simulink model "bandpass_eq"  (R2023a)
settings: Solver=FixedStepDiscrete  StartTime=0.0  StopTime=simParams.stopTime  RelTol=1e-3
PostLoadFcn:
  | postLoadCallback
InitFcn:
  | initCallback
StopFcn:
  | stopCallback
values from neighbouring files (symbols this model uses):
  modelParams = createFFTFilters(modelParams)    [createModelParams.m]
libraries: hdlsllib x13, dspsrcs4 x7, simulink x7, dsphdlxfrm2 x2, dspsigops x1
CloseFcn:
  | closeCallback
settings Model: DataTypeOverride=Off  Creator=Ross  LastModifiedBy=Antho
settings SolverCC: AlgebraicLoopSolver=TrustRegion
settings DataIOCC: ReturnWorkspaceOutputs=off
settings OptimizationCC: BlockReduction=off  ConditionallyExecuteInputs=off  DefaultParameterBehavior=Inlined  InheritOutputTypeSmallerThanSingle=on
settings DebuggingCC: ReadBeforeWriteMsg=DisableAll  WriteAfterWriteMsg=DisableAll  WriteAfterReadMsg=DisableAll  AlgebraicLoopMsg=error  MultiTaskDSMMsg=none  SingleTaskRateTransMsg=error  UnconnectedInputMsg=warning  UnconnectedOutputMsg=warning  UnconnectedLineMsg=warning  PregeneratedLibrarySubsystemCodeDiagnostic=none  ArithmeticOperatorsInVariantConditions=warning
settings HardwareCC: ProdBitPerPointer=32  ProdBitPerSizeT=32  ProdBitPerPtrDiffT=32  ProdLargestAtomicFloat=None  ProdIntDivRoundTo=Undefined  ProdEndianess=Unspecified  ProdWordSize=32  ProdHWDeviceType=ASIC/FPGA->ASIC/FPGA  TargetBitPerPointer=64  TargetBitPerSizeT=64  TargetBitPerPtrDiffT=64  TargetLongLongMode=on  TargetIntDivRoundTo=Zero  TargetEndianess=LittleEndian  TargetWordSize=64  TargetHWDeviceType=Custom Processor->MATLAB Host Computer  ProdEqTarget=off
settings ModelReferenceCC: UpdateModelReferenceTargets=IfOutOfDate  EnableRefExpFcnMdlSchedulingChecks=on
settings SFSimCC: SFSimEcho=off  SimUseLocalCustomCode=off  CustomCodeUndefinedFunction=UseInterfaceOnly
settings RTWCC: RTWUseLocalCustomCode=off  DLArmComputeVersion=19.05

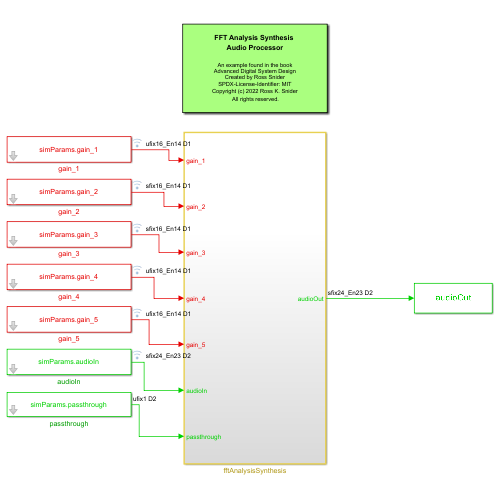
[thumbnail: Simulink's stored preview of the top-level diagram]
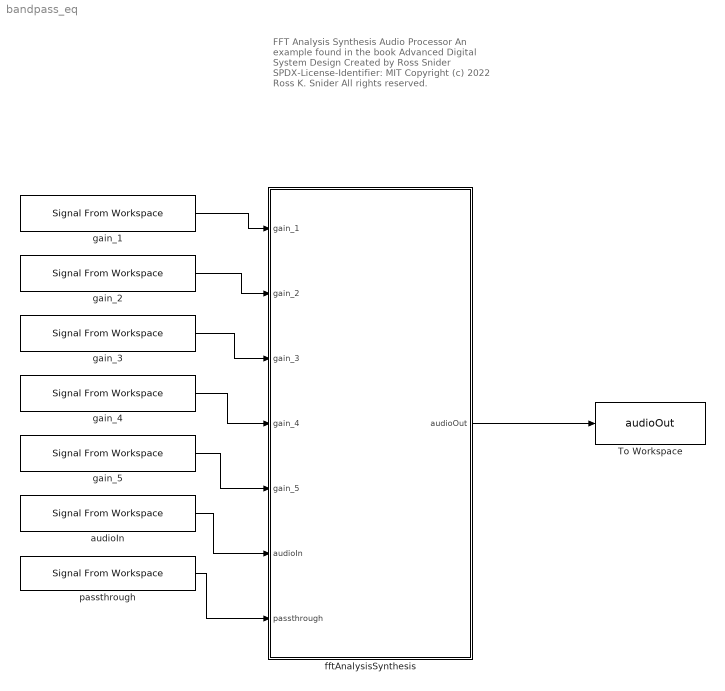
== system bandpass_eq ==
  note: FFT Analysis Synthesis
      | Audio Processor
      |
      | An example found in the book
      | Advanced Digital System Design
      | Created by Ross Snider
      | SPDX-License-Identifier: MIT
      | Copyright (c) 2022 Ross K. Snider
      | All rights reserved.
  To Workspace : ToWorkspace  VariableName=audioOut  SampleTime=-1
      settings: Save2DSignal=2-D array (concatenate along first dimension)
  audioIn : dspsrcs4/Signal From Workspace  X=simParams.audioIn  Ts=modelParams.audio.samplePeriod  nsamps=1  OutputAfterFinalValue=Setting to zero  ignoreOrWarnInputAndFrameLengths=off  OutputFrames=off
  fftAnalysisSynthesis : Subsystem  TreatAsAtomicUnit=on
  gain_1 : dspsrcs4/Signal From Workspace  X=simParams.gain_1  Ts=modelParams.audio.samplePeriod/modelParams.system.upsampleFactor  nsamps=1  OutputAfterFinalValue=Holding final value  ignoreOrWarnInputAndFrameLengths=off  OutputFrames=off
  gain_2 : dspsrcs4/Signal From Workspace  X=simParams.gain_2  Ts=modelParams.audio.samplePeriod/modelParams.system.upsampleFactor  nsamps=1  OutputAfterFinalValue=Holding final value  ignoreOrWarnInputAndFrameLengths=off  OutputFrames=off
  gain_3 : dspsrcs4/Signal From Workspace  X=simParams.gain_3  Ts=modelParams.audio.samplePeriod/modelParams.system.upsampleFactor  nsamps=1  OutputAfterFinalValue=Holding final value  ignoreOrWarnInputAndFrameLengths=off  OutputFrames=off
  gain_4 : dspsrcs4/Signal From Workspace  X=simParams.gain_4  Ts=modelParams.audio.samplePeriod/modelParams.system.upsampleFactor  nsamps=1  OutputAfterFinalValue=Holding final value  ignoreOrWarnInputAndFrameLengths=off  OutputFrames=off
  gain_5 : dspsrcs4/Signal From Workspace  X=simParams.gain_5  Ts=modelParams.audio.samplePeriod/modelParams.system.upsampleFactor  nsamps=1  OutputAfterFinalValue=Holding final value  ignoreOrWarnInputAndFrameLengths=off  OutputFrames=off
  passthrough : dspsrcs4/Signal From Workspace  X=simParams.passthrough  Ts=modelParams.audio.samplePeriod  nsamps=1  OutputAfterFinalValue=Holding final value  ignoreOrWarnInputAndFrameLengths=off  OutputFrames=off
  wires:
  fftAnalysisSynthesis/1(audioOut) -> To Workspace/1
  audioIn/1 -> fftAnalysisSynthesis/6(audioIn)
  passthrough/1 -> fftAnalysisSynthesis/7(passthrough)
  gain_5/1 -> fftAnalysisSynthesis/5(gain_5)
  gain_4/1 -> fftAnalysisSynthesis/4(gain_4)
  gain_3/1 -> fftAnalysisSynthesis/3(gain_3)
  gain_2/1 -> fftAnalysisSynthesis/2(gain_2)
  gain_1/1 -> fftAnalysisSynthesis/1(gain_1)

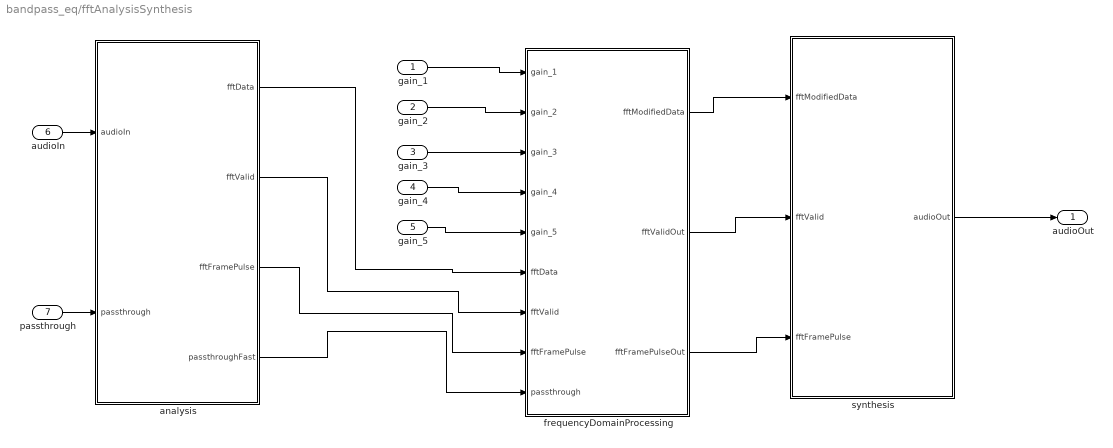
== system bandpass_eq/fftAnalysisSynthesis ==
  gain_1 : Inport
  gain_2 : Inport  Port=2
  gain_3 : Inport  Port=3
  gain_4 : Inport  Port=4
  gain_5 : Inport  Port=5
  audioIn : Inport  Port=6
  passthrough : Inport  Port=7
  analysis : Subsystem
  frequencyDomainProcessing : Subsystem
  synthesis : Subsystem
  audioOut : Outport  VectorParamsAs1DForOutWhenUnconnected=off
  wires:
  audioIn/1 -> analysis/1(audioIn)
  synthesis/1(audioOut) -> audioOut/1
  analysis/1(fftData) -> frequencyDomainProcessing/6(fftData)
  analysis/2(fftValid) -> frequencyDomainProcessing/7(fftValid)
  analysis/3(fftFramePulse) -> frequencyDomainProcessing/8(fftFramePulse)
  frequencyDomainProcessing/1(fftModifiedData) -> synthesis/1(fftModifiedData)
  frequencyDomainProcessing/2(fftValidOut) -> synthesis/2(fftValid)
  frequencyDomainProcessing/3(fftFramePulseOut) -> synthesis/3(fftFramePulse)
  analysis/4(passthroughFast) -> frequencyDomainProcessing/9(passthrough)
  passthrough/1 -> analysis/2(passthrough)
  gain_5/1 -> frequencyDomainProcessing/5(gain_5)
  gain_4/1 -> frequencyDomainProcessing/4(gain_4)
  gain_3/1 -> frequencyDomainProcessing/3(gain_3)
  gain_2/1 -> frequencyDomainProcessing/2(gain_2)
  gain_1/1 -> frequencyDomainProcessing/1(gain_1)

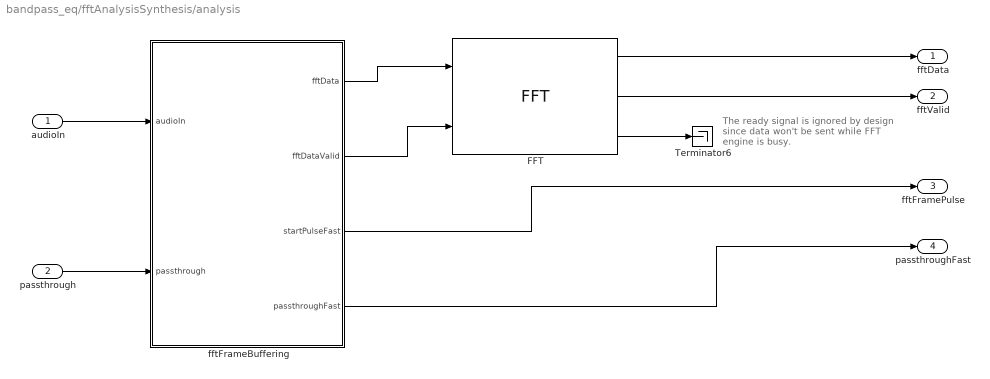
== system bandpass_eq/fftAnalysisSynthesis/analysis ==
  note: The ready signal is ignored by design
      | since data won't be sent while FFT
      | engine is busy.
  audioIn : Inport
  passthrough : Inport  Port=2
  FFT : dsphdlxfrm2/FFT  FFTLength=modelParams.fft.size  Architecture=Burst Radix 2  ComplexMultiplication=Use 4 multipliers and 2 adders  BitReversedOutput=off  BitReversedInput=off  Normalize=off  SimulateUsing=Code generation  RoundingMethod=Floor  ResetInputPort=off  StartOutputPort=off  EndOutputPort=off
  Terminator6 : Terminator
  fftFrameBuffering : Subsystem
  fftData : Outport  VectorParamsAs1DForOutWhenUnconnected=off
  fftValid : Outport  Port=2  VectorParamsAs1DForOutWhenUnconnected=off
  fftFramePulse : Outport  Port=3  VectorParamsAs1DForOutWhenUnconnected=off
  passthroughFast : Outport  Port=4
  wires:
  FFT/3 -> Terminator6/1
  fftFrameBuffering/3(startPulseFast) -> fftFramePulse/1
  audioIn/1 -> fftFrameBuffering/1(audioIn)
  fftFrameBuffering/2(fftDataValid) -> FFT/2
  fftFrameBuffering/1(fftData) -> FFT/1
  FFT/1 -> fftData/1
  FFT/2 -> fftValid/1
  fftFrameBuffering/4(passthroughFast) -> passthroughFast/1
  passthrough/1 -> fftFrameBuffering/2(passthrough)

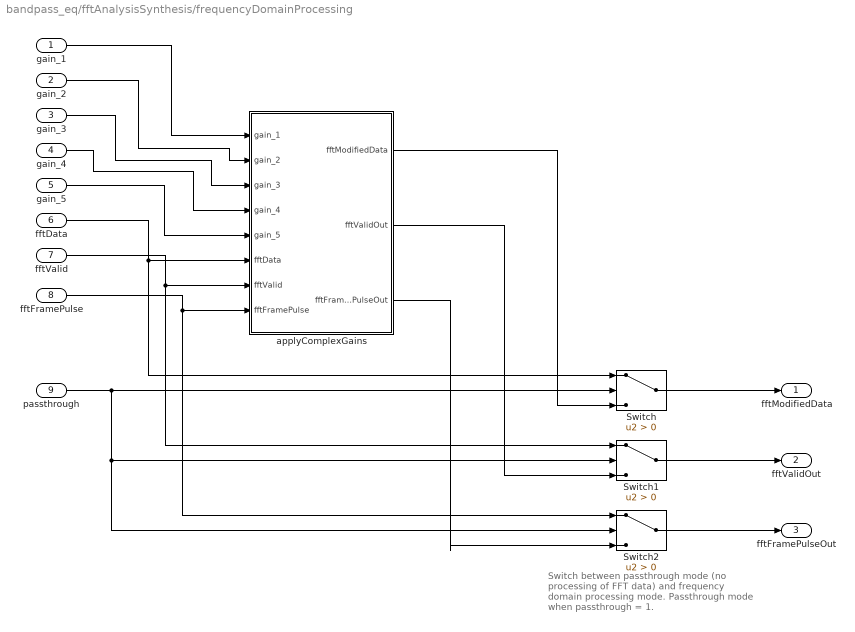
== system bandpass_eq/fftAnalysisSynthesis/frequencyDomainProcessing ==
  note: Switch between passthrough mode
      | (no processing of FFT data)
      | and frequency domain processing mode.
      | Passthrough mode when passthrough = 1.
  gain_1 : Inport
  gain_2 : Inport  Port=2
  gain_3 : Inport  Port=3
  gain_4 : Inport  Port=4
  gain_5 : Inport  Port=5
  fftData : Inport  Port=6
  fftValid : Inport  Port=7
  fftFramePulse : Inport  Port=8
  passthrough : Inport  Port=9
  Switch : Switch  Criteria=u2 > Threshold  SaturateOnIntegerOverflow=off  InputSameDT=off
  Switch1 : Switch  Criteria=u2 > Threshold  SaturateOnIntegerOverflow=off  InputSameDT=off
  Switch2 : Switch  Criteria=u2 > Threshold  SaturateOnIntegerOverflow=off  InputSameDT=off
  applyComplexGains : Subsystem
  fftModifiedData : Outport  VectorParamsAs1DForOutWhenUnconnected=off
  fftValidOut : Outport  Port=2  VectorParamsAs1DForOutWhenUnconnected=off
  fftFramePulseOut : Outport  Port=3
  wires:
  fftData/1 -> Switch/1, applyComplexGains/6(fftData)
  fftValid/1 -> Switch1/1, applyComplexGains/7(fftValid)
  applyComplexGains/1(fftModifiedData) -> Switch/3
  applyComplexGains/2(fftValidOut) -> Switch1/3
  fftFramePulse/1 -> Switch2/1, applyComplexGains/8(fftFramePulse)
  passthrough/1 -> Switch2/2, Switch1/2, Switch/2
  Switch/1 -> fftModifiedData/1
  applyComplexGains/3(fftFramePulseOut) -> Switch2/3
  Switch1/1 -> fftValidOut/1
  Switch2/1 -> fftFramePulseOut/1
  gain_1/1 -> applyComplexGains/1(gain_1)
  gain_2/1 -> applyComplexGains/2(gain_2)
  gain_3/1 -> applyComplexGains/3(gain_3)
  gain_4/1 -> applyComplexGains/4(gain_4)
  gain_5/1 -> applyComplexGains/5(gain_5)

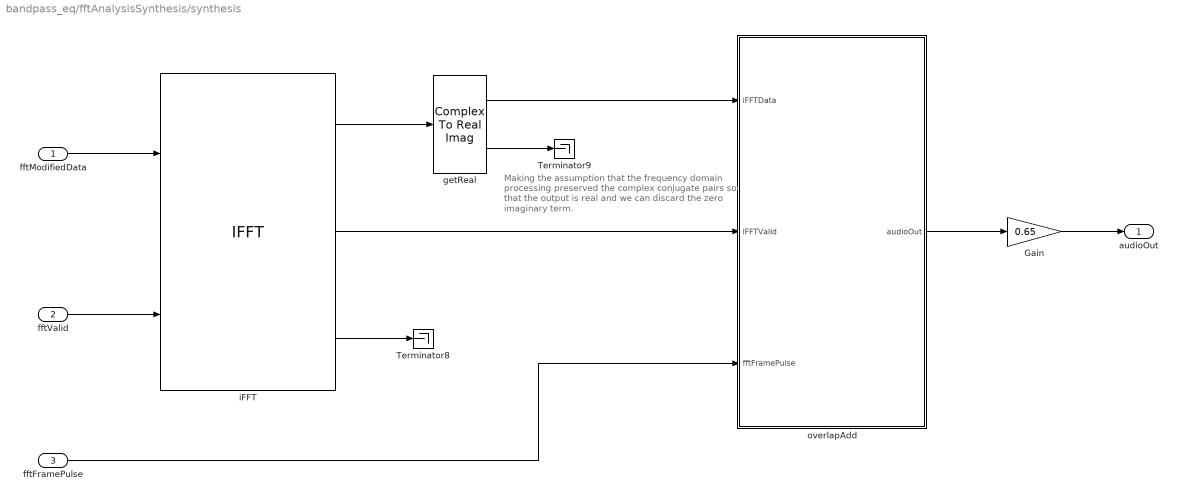
== system bandpass_eq/fftAnalysisSynthesis/synthesis ==
  note: Making the assumption that the frequency domain processing preserved the complex conjugate pairs so that the output is real and we can discard the zero imaginary term.
  fftModifiedData : Inport
  fftValid : Inport  Port=2
  fftFramePulse : Inport  Port=3
  Gain : Gain  Gain=0.65  OutDataTypeStr=modelParams.audio.dataType
  Terminator8 : Terminator
  Terminator9 : Terminator
  getReal : ComplexToRealImag
  iFFT : dsphdlxfrm2/IFFT  FFTLength=modelParams.fft.size  Architecture=Burst Radix 2  ComplexMultiplication=Use 4 multipliers and 2 adders  BitReversedOutput=off  BitReversedInput=off  Normalize=on  SimulateUsing=Code generation  RoundingMethod=Floor  ResetInputPort=off  StartOutputPort=off  EndOutputPort=off
  overlapAdd : Subsystem
  audioOut : Outport  VectorParamsAs1DForOutWhenUnconnected=off
  wires:
  iFFT/3 -> Terminator8/1
  iFFT/2 -> overlapAdd/2(iFFTValid)
  getReal/1 -> overlapAdd/1(iFFTData)
  fftModifiedData/1 -> iFFT/1
  overlapAdd/1(audioOut) -> Gain/1
  iFFT/1 -> getReal/1
  getReal/2 -> Terminator9/1
  fftValid/1 -> iFFT/2
  fftFramePulse/1 -> overlapAdd/3(fftFramePulse)
  Gain/1 -> audioOut/1

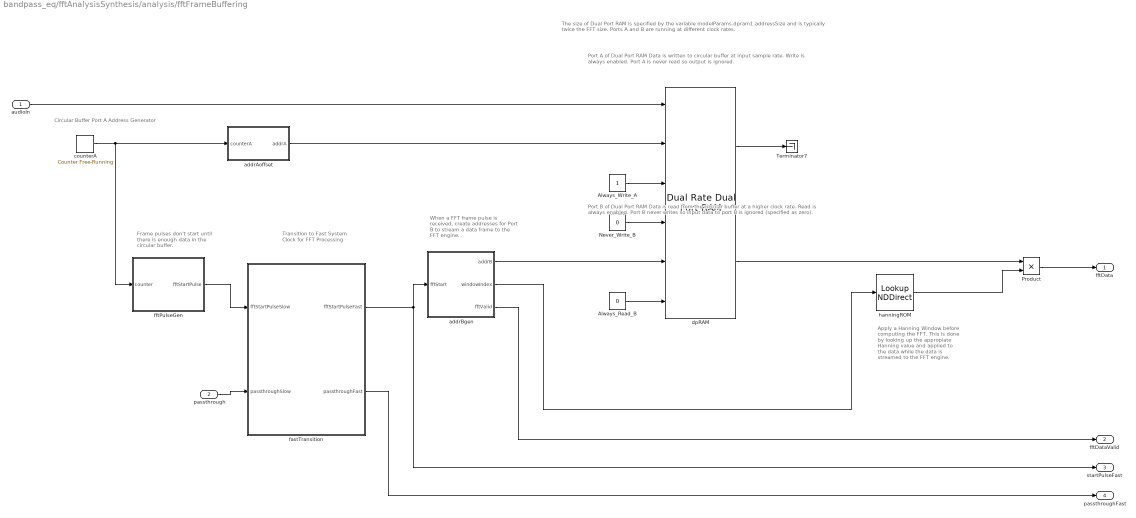
== system bandpass_eq/fftAnalysisSynthesis/analysis/fftFrameBuffering ==
  note: When a FFT frame pulse
      | is received, create addresses for
      | Port B to stream a data frame
      | to the FFT engine.
  note: Apply a Hanning Window
      | before computing the FFT.
      | This is done by looking up
      | the appropiate Hanning value
      | and applied to the data while
      | the data is streamed to the
      | FFT engine.
  note: Frame pulses don't start
      | until there is enough data
      | in the circular buffer.
  note: The size of Dual Port RAM is specified by the variable
      | modelParams.dpram1.addressSize  and is typically twice the FFT size.
      | Ports A and B are running at different clock rates.
  note: Circular Buffer
      | Port A Address Generator
  note: Port A of Dual Port RAM
      |
      | Data is written to circular buffer at input sample rate.
      | Write is always enabled.  Port A is never read so output is ignored.
  note: Transition to
      | Fast System Clock
      | for FFT Processing
  note: Port B of Dual Port RAM
      |
      | Data is read from the circular buffer at a higher clock rate.
      | Read is always enabled.  Port B never writes so input data to port B
      | is ignored (specified as zero).
  audioIn : Inport
  passthrough : Inport  Port=2
  Always_Read_B : Constant  Value=0  OutDataTypeStr=boolean  SampleTime=modelParams.audio.samplePeriod/modelParams.system.upsampleFactor
  Always_Write_A : Constant  OutDataTypeStr=boolean  SampleTime=modelParams.audio.samplePeriod
  Never_Write_B : Constant  Value=0  OutDataTypeStr=modelParams.audio.dataType  SampleTime=modelParams.audio.samplePeriod/modelParams.system.upsampleFactor
  Product : Product  OutDataTypeStr=modelParams.audio.dataType
  Terminator7 : Terminator
  addrAoffset : Subsystem
  addrBgen : Subsystem
  counterA : simulink/Sources/Counter Free-Running  NumBits=modelParams.dpram1.addressSize  tsamp=modelParams.audio.samplePeriod
  dpRAM : hdlsllib/HDL RAMs/Dual Rate Dual Port RAM  ram_size=modelParams.dpram1.addressSize
  fastTransition : Subsystem
  fftPulseGen : Subsystem
  hanningROM : LookupNDDirect  NumberOfTableDimensions=1  Table=modelParams.hanningWindow.coefficients
  fftData : Outport  VectorParamsAs1DForOutWhenUnconnected=off
  fftDataValid : Outport  Port=2  VectorParamsAs1DForOutWhenUnconnected=off
  startPulseFast : Outport  Port=3  VectorParamsAs1DForOutWhenUnconnected=off
  passthroughFast : Outport  Port=4
  wires:
  Always_Write_A/1 -> dpRAM/3
  Never_Write_B/1 -> dpRAM/4
  Always_Read_B/1 -> dpRAM/6
  dpRAM/1 -> Terminator7/1
  counterA/1 -> addrAoffset/1(counterA), fftPulseGen/1(counter)
  audioIn/1 -> dpRAM/1
  addrAoffset/1(addrA) -> dpRAM/2
  dpRAM/2 -> Product/1
  Product/1 -> fftData/1
  fastTransition/1(fftStartPulseFast) -> addrBgen/1(fftStart), startPulseFast/1
  fftPulseGen/1(fftStartPulse) -> fastTransition/1(fftStartPulseSlow)
  addrBgen/3(fftValid) -> fftDataValid/1
  passthrough/1 -> fastTransition/2(passthroughSlow)
  fastTransition/2(passthroughFast) -> passthroughFast/1
  addrBgen/1(addrB) -> dpRAM/5
  addrBgen/2(windowIndex) -> hanningROM/1
  hanningROM/1 -> Product/2

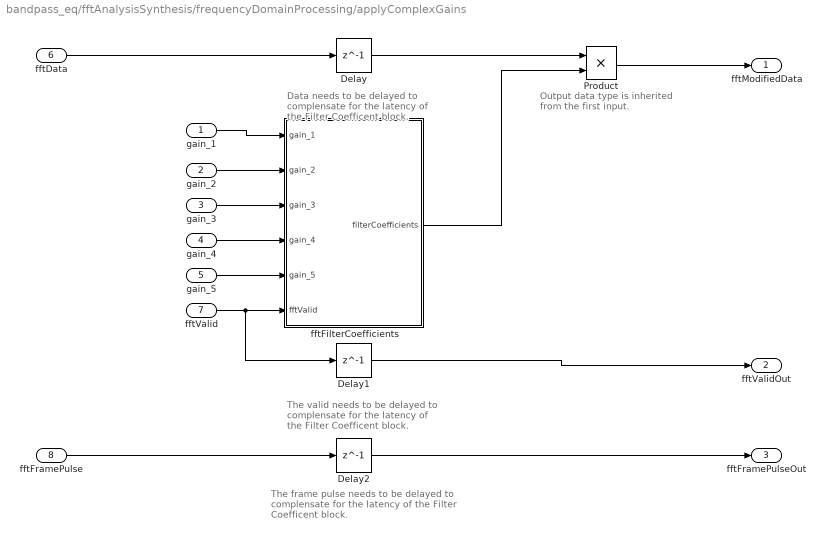
== system bandpass_eq/fftAnalysisSynthesis/frequencyDomainProcessing/applyComplexGains ==
  note: Output data type is inherited
      | from the first input.
  note: The frame pulse needs to be delayed
      | to complensate for the latency
      | of the Filter Coefficent block.
  note: The valid needs to be delayed
      | to complensate for the latency
      | of the Filter Coefficent block.
  note: Data needs to be delayed
      | to complensate for the latency
      | of the Filter Coefficent block.
  gain_1 : Inport
  gain_2 : Inport  Port=2
  gain_3 : Inport  Port=3
  gain_4 : Inport  Port=4
  gain_5 : Inport  Port=5
  fftData : Inport  Port=6
  fftValid : Inport  Port=7
  fftFramePulse : Inport  Port=8
  Delay : Delay  DelayLength=1
  Delay1 : Delay  DelayLength=1
  Delay2 : Delay  DelayLength=1
  Product : Product  OutDataTypeStr=Inherit: Same as first input
  fftFilterCoefficients : Subsystem
  fftModifiedData : Outport
  fftValidOut : Outport  Port=2
  fftFramePulseOut : Outport  Port=3
  wires:
  fftValid/1 -> Delay1/1, fftFilterCoefficients/6(fftValid)
  fftData/1 -> Delay/1
  fftFramePulse/1 -> Delay2/1
  Delay2/1 -> fftFramePulseOut/1
  fftFilterCoefficients/1(filterCoefficients) -> Product/2
  Product/1 -> fftModifiedData/1
  Delay1/1 -> fftValidOut/1
  Delay/1 -> Product/1
  gain_1/1 -> fftFilterCoefficients/1(gain_1)
  gain_2/1 -> fftFilterCoefficients/2(gain_2)
  gain_3/1 -> fftFilterCoefficients/3(gain_3)
  gain_4/1 -> fftFilterCoefficients/4(gain_4)
  gain_5/1 -> fftFilterCoefficients/5(gain_5)

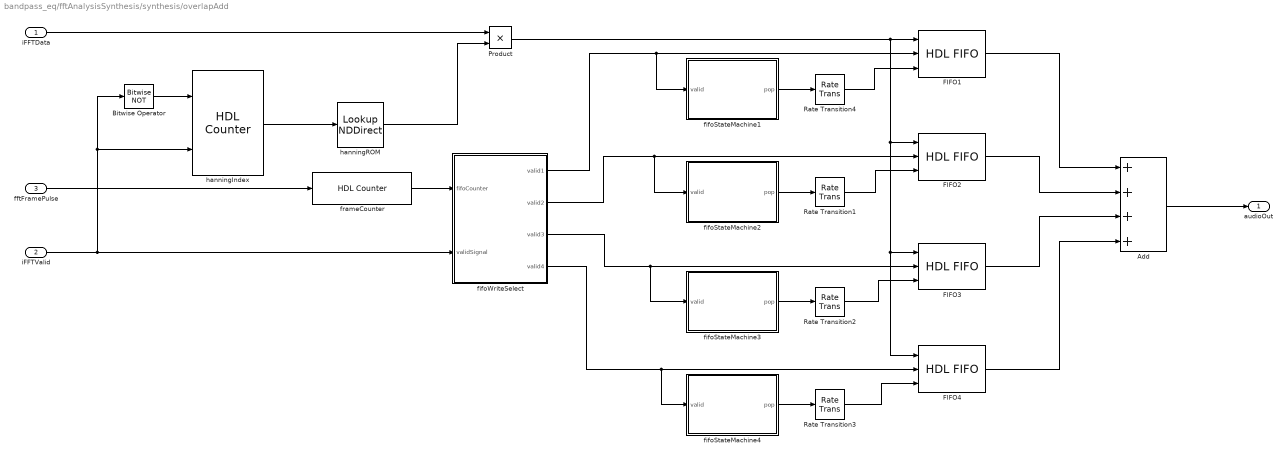
== system bandpass_eq/fftAnalysisSynthesis/synthesis/overlapAdd ==
  iFFTData : Inport
  iFFTValid : Inport  Port=2
  fftFramePulse : Inport  Port=3
  Add : Sum  Inputs=4
  Bitwise Operator : simulink/Logic and Bit Operations/Bitwise Operator  logicop=NOT  UseBitMask=off  BitMask=bin2dec('11011001')  BitMaskRealWorld=Stored Integer
  FIFO{1..4} (4 alike) : hdlsllib/HDL RAMs/HDL FIFO  fifo_size=modelParams.fft.size  mode=Classic  ratio=modelParams.system.upsampleFactor  push_msg=Warning  pop_msg=Warning  show_empty=off  show_full=off  show_num=off  LabelModeActiveChoice_Mode=Classic  rst_port=off
  Product : Product  OutDataTypeStr=Inherit: Same as first input
  Rate Transition{1..4} (4 alike) : RateTransition  OutPortSampleTimeOpt=Multiple of input port sample time  OutPortSampleTimeMultiple=modelParams.system.upsampleFactor
  fifoStateMachine1 : MATLAB Function  TreatAsAtomicUnit=on
  fifoStateMachine2 : MATLAB Function  TreatAsAtomicUnit=on
  fifoStateMachine3 : MATLAB Function  TreatAsAtomicUnit=on
  fifoStateMachine4 : MATLAB Function  TreatAsAtomicUnit=on
  fifoWriteSelect : MATLAB Function  TreatAsAtomicUnit=on
  frameCounter : hdlsllib/Sources/HDL Counter  CountType=Free running  CountInit=2  CountStep=1  CountMax=1024  CountFromType=Initial value  CountFrom=2  CountResetPort=off  CountLoadPort=off  CountEnbPort=on  CountDirPort=off  CountHitOutputPort=off  CountDataType=Unsigned  CountWordLen=2  CountFracLen=0  CountSampTime=1
  hanningIndex : hdlsllib/Sources/HDL Counter  CountType=Count limited  CountInit=0  CountStep=1  CountMax=modelParams.fft.size  CountFromType=Initial value  CountFrom=0  CountResetPort=on  CountLoadPort=off  CountEnbPort=on  CountDirPort=off  CountHitOutputPort=off  CountDataType=Unsigned  CountWordLen=modelParams.dpram1.addressSize  CountFracLen=0  CountSampTime=1
  hanningROM : LookupNDDirect  NumberOfTableDimensions=1  Table=modelParams.hanningWindow.coefficients
  audioOut : Outport  VectorParamsAs1DForOutWhenUnconnected=off
  wires:
  FIFO1/1 -> Add/1
  FIFO3/1 -> Add/3
  fftFramePulse/1 -> frameCounter/1
  FIFO2/1 -> Add/2
  fifoWriteSelect/3(valid3) -> fifoStateMachine3/1(valid), FIFO3/2
  fifoWriteSelect/4(valid4) -> fifoStateMachine4/1(valid), FIFO4/2
  FIFO4/1 -> Add/4
  fifoWriteSelect/1(valid1) -> fifoStateMachine1/1(valid), FIFO1/2
  fifoWriteSelect/2(valid2) -> fifoStateMachine2/1(valid), FIFO2/2
  Add/1 -> audioOut/1
  frameCounter/1 -> fifoWriteSelect/1(fifoCounter)
  Bitwise Operator/1 -> hanningIndex/1
  iFFTValid/1 -> hanningIndex/2, Bitwise Operator/1, fifoWriteSelect/2(validSignal)
  iFFTData/1 -> Product/1
  hanningROM/1 -> Product/2
  hanningIndex/1 -> hanningROM/1
  fifoStateMachine1/1(pop) -> Rate Transition4/1
  Rate Transition4/1 -> FIFO1/3
  fifoStateMachine2/1(pop) -> Rate Transition1/1
  Rate Transition1/1 -> FIFO2/3
  fifoStateMachine3/1(pop) -> Rate Transition2/1
  Rate Transition2/1 -> FIFO3/3
  fifoStateMachine4/1(pop) -> Rate Transition3/1
  Rate Transition3/1 -> FIFO4/3
  Product/1 -> FIFO3/1, FIFO4/1, FIFO2/1, FIFO1/1

== system bandpass_eq/fftAnalysisSynthesis/analysis/fftFrameBuffering/addrAoffset ==
  note: Adding 1 to counter since the read pointer (addr_B) can catch the write pointer (addr_A)
      | if modelParams.system.upsampleFactor is large enough and Simulink will throw an error.
      | It would be nice if the HDL Coder allowed a read-before-write option when
      | the addresses are identical, which some memories support.
  counterA : Inport
  Add : Sum  OutDataTypeStr=fixdt(0,modelParams.dpram1.addressSize,0)
  writeOffset : Constant  OutDataTypeStr=fixdt(0,modelParams.dpram1.addressSize,0)  SampleTime=modelParams.audio.samplePeriod
  addrA : Outport  VectorParamsAs1DForOutWhenUnconnected=off
  wires:
  writeOffset/1 -> Add/2
  Add/1 -> addrA/1
  counterA/1 -> Add/1

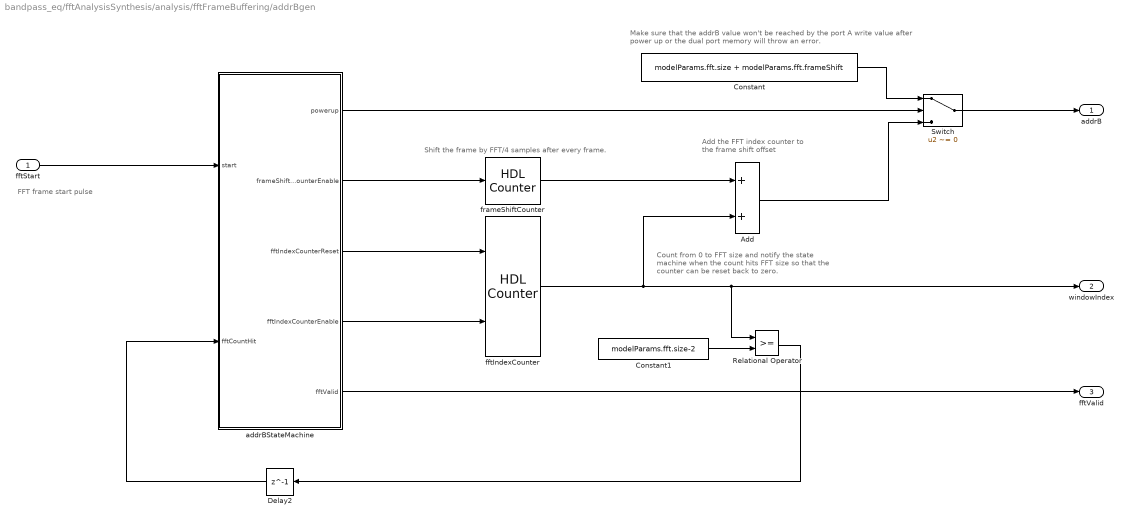
== system bandpass_eq/fftAnalysisSynthesis/analysis/fftFrameBuffering/addrBgen ==
  note: Shift the frame by FFT/4 samples after every frame.
  note: Count from 0 to FFT size and notify the
      | state machine when the count hits FFT size
      | so that the counter can be reset back to zero.
  note: Add the FFT index counter to
      | the frame shift offset
  note: FFT frame start pulse
  note: Make sure that the addrB value won't be reached by the port A
      | write value after power up or the dual port memory will throw an error.
  fftStart : Inport
  Add : Sum  OutDataTypeStr=fixdt(0,modelParams.dpram1.addressSize,0)
  Constant : Constant  Value=modelParams.fft.size + modelParams.fft.frameShift  OutDataTypeStr=fixdt(0,modelParams.dpram1.addressSize,0)  SampleTime=modelParams.audio.samplePeriod/modelParams.system.upsampleFactor
  Constant1 : Constant  Value=modelParams.fft.size-2  OutDataTypeStr=fixdt(0,modelParams.dpram1.addressSize,0)  SampleTime=modelParams.audio.samplePeriod/modelParams.system.upsampleFactor
  Delay2 : Delay  DelayLength=1
  Relational Operator : RelationalOperator  OutDataTypeStr=boolean  RndMeth=Simplest  InputSameDT=off
  Switch : Switch  Criteria=u2 ~= 0  SaturateOnIntegerOverflow=off  InputSameDT=off
  addrBStateMachine : MATLAB Function  TreatAsAtomicUnit=on
  fftIndexCounter : hdlsllib/Sources/HDL Counter  CountType=Free running  CountInit=0  CountStep=1  CountMax=modelParams.fft.size-1  CountFromType=Initial value  CountFrom=0  CountResetPort=on  CountLoadPort=off  CountEnbPort=on  CountDirPort=off  CountHitOutputPort=off  CountDataType=Unsigned  CountWordLen=modelParams.dpram1.addressSize  CountFracLen=0  CountSampTime=1
  frameShiftCounter : hdlsllib/Sources/HDL Counter  CountType=Free running  CountInit=0  CountStep=modelParams.fft.frameShift  CountMax=modelParams.fft.size  CountFromType=Initial value  CountFrom=0  CountResetPort=off  CountLoadPort=off  CountEnbPort=on  CountDirPort=off  CountHitOutputPort=off  CountDataType=Unsigned  CountWordLen=modelParams.dpram1.addressSize  CountFracLen=0  CountSampTime=1
  addrB : Outport
  windowIndex : Outport  Port=2
  fftValid : Outport  Port=3
  wires:
  Relational Operator/1 -> Delay2/1
  Switch/1 -> addrB/1
  Add/1 -> Switch/3
  Constant/1 -> Switch/1
  addrBStateMachine/1(powerup) -> Switch/2
  frameShiftCounter/1 -> Add/1
  addrBStateMachine/3(fftIndexCounterReset) -> fftIndexCounter/1
  addrBStateMachine/2(frameShiftCounterEnable) -> frameShiftCounter/1
  fftIndexCounter/1 -> Add/2, Relational Operator/1, windowIndex/1
  fftStart/1 -> addrBStateMachine/1(start)
  addrBStateMachine/5(fftValid) -> fftValid/1
  addrBStateMachine/4(fftIndexCounterEnable) -> fftIndexCounter/2
  Delay2/1 -> addrBStateMachine/2(fftCountHit)
  Constant1/1 -> Relational Operator/2

== system bandpass_eq/fftAnalysisSynthesis/analysis/fftFrameBuffering/fastTransition ==
  note: The upsample block inserts zeros between samples.
      | We want the pulse that is only one clock period wide at the
      | faster clock rate, so inserting zeros is what we want.
  note: The rate transition block registers and keeps the same
      | value. We want the enable signal to always be enabled,
      | so keeping the same value using the unit delay is what we want.
  note: Transition Signals to Fast System Clock Rate
      | We need to be careful whether we are
      | 1. Inserting zeros
      | or
      | 2. Keeping the same value
  fftStartPulseSlow : Inport
  passthroughSlow : Inport  Port=2
  Rate Transition1 : RateTransition  OutPortSampleTimeOpt=Multiple of input port sample time  OutPortSampleTimeMultiple=1/modelParams.system.upsampleFactor
  Upsample : dspsigops/Upsample  FactorSource=Dialog parameter  N=modelParams.system.upsampleFactor  Nmax=16  phase=0  RateOptions=Allow multirate processing  ic=0  mode=Unused parameter value
  fftStartPulseFast : Outport
  passthroughFast : Outport  Port=2
  wires:
  fftStartPulseSlow/1 -> Upsample/1
  Upsample/1 -> fftStartPulseFast/1
  passthroughSlow/1 -> Rate Transition1/1
  Rate Transition1/1 -> passthroughFast/1

== system bandpass_eq/fftAnalysisSynthesis/analysis/fftFrameBuffering/fftPulseGen ==
  note: Don't send out FFT frame start pulses
      | until circular buffer has filled.
  counter : Inport
  fftFramePulseGen : Subsystem
  waitForData : Subsystem
  fftStartPulse : Outport  VectorParamsAs1DForOutWhenUnconnected=off
  wires:
  counter/1 -> fftFramePulseGen/1("counterValue ")
  waitForData/1(fftFramePulse) -> fftStartPulse/1
  fftFramePulseGen/1(framePulse) -> waitForData/1(framePulse)

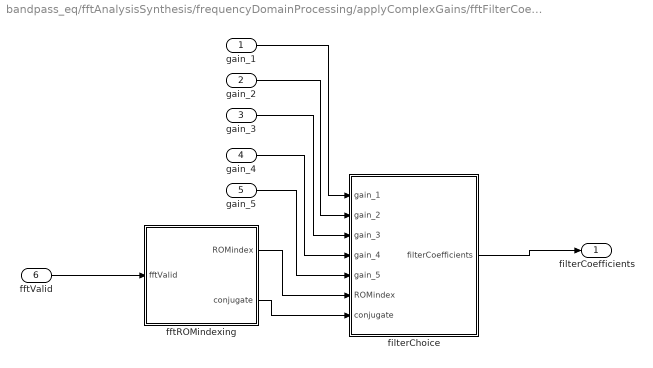
== system bandpass_eq/fftAnalysisSynthesis/frequencyDomainProcessing/applyComplexGains/fftFilterCoefficients ==
  gain_1 : Inport
  gain_2 : Inport  Port=2
  gain_3 : Inport  Port=3
  gain_4 : Inport  Port=4
  gain_5 : Inport  Port=5
  fftValid : Inport  Port=6
  fftROMindexing : Subsystem
  filterChoice : Subsystem
  filterCoefficients : Outport
  wires:
  fftROMindexing/1(ROMindex) -> filterChoice/6(ROMindex)
  fftValid/1 -> fftROMindexing/1(fftValid)
  filterChoice/1(filterCoefficients) -> filterCoefficients/1
  fftROMindexing/2(conjugate) -> filterChoice/7(conjugate)
  gain_1/1 -> filterChoice/1(gain_1)
  gain_2/1 -> filterChoice/2(gain_2)
  gain_3/1 -> filterChoice/3(gain_3)
  gain_4/1 -> filterChoice/4(gain_4)
  gain_5/1 -> filterChoice/5(gain_5)

== system bandpass_eq/fftAnalysisSynthesis/analysis/fftFrameBuffering/fftPulseGen/fftFramePulseGen ==
  note: Create a FFT frame pulse that happens every FFT_size/4 samples.
      | We do this by watching when an appropriate subset of the counter bits
      | become zero.
  "counterValue " : Inport
  Bit Slice : hdlsllib/Logic and Bit Operations/Bit Slice  lidx=modelParams.fft.frameShiftNbits-1  ridx=0
  Compare To Zero : simulink/Logic and Bit Operations/Compare To Zero  relop===  OutDataTypeStr=boolean
  framePulse : Outport  VectorParamsAs1DForOutWhenUnconnected=off
  wires:
  "counterValue "/1 -> Bit Slice/1
  Compare To Zero/1 -> framePulse/1
  Bit Slice/1 -> Compare To Zero/1

== system bandpass_eq/fftAnalysisSynthesis/analysis/fftFrameBuffering/fftPulseGen/waitForData ==
  note: Frame pulses don't start
      | coming through until
      | circular buffer has data.
  note: Counter starts a zero and counts number of frame pulses.
      | Counter remains enabled while frame count is less than 4.
      | As soon as the counter reaches 4, it is disabled, which then
      | enables the frame pulses to pass through.
  note: framePulse
      | will pass through
      | when enabled
  note: Number of Frames
      | to wait before starting
  note: Start performing FFTs after enough data has filled the circular buffer.
      | This is due to the fact that we don't want the read pointer (addrB)
      | to catch up with the write pointer (addrA) because if it does,
      | the dpRAM will throw an assertion error.
  framePulse : Inport
  Bitwise Operator : simulink/Logic and Bit Operations/Bitwise Operator  logicop=NOT  UseBitMask=off  BitMask=bin2dec('11011001')  BitMaskRealWorld=Stored Integer
  Compare To Constant : simulink/Logic and Bit Operations/Compare To Constant  relop=<  const=4  OutDataTypeStr=boolean
  Logical Operator : Logic  AllPortsSameDT=off  OutDataTypeStr=boolean
  Logical Operator1 : Logic  AllPortsSameDT=off  OutDataTypeStr=boolean
  initialFrameCount : hdlsllib/Sources/HDL Counter  CountType=Count limited  CountInit=0  CountStep=1  CountMax=4  CountFromType=Specify  CountFrom=0  CountResetPort=off  CountLoadPort=off  CountEnbPort=on  CountDirPort=off  CountHitOutputPort=off  CountDataType=Unsigned  CountWordLen=5  CountFracLen=0  CountSampTime=1
  fftFramePulse : Outport  VectorParamsAs1DForOutWhenUnconnected=off
  wires:
  Logical Operator1/1 -> fftFramePulse/1
  framePulse/1 -> Logical Operator/2, Logical Operator1/1
  initialFrameCount/1 -> Compare To Constant/1
  Logical Operator/1 -> initialFrameCount/1
  Compare To Constant/1 -> Bitwise Operator/1, Logical Operator/1
  Bitwise Operator/1 -> Logical Operator1/2

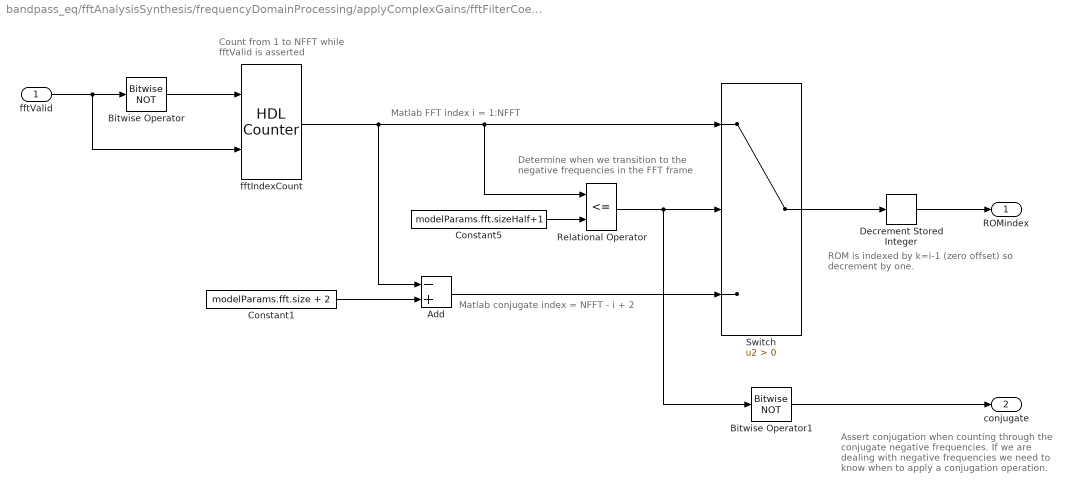
== system bandpass_eq/fftAnalysisSynthesis/frequencyDomainProcessing/applyComplexGains/fftFilterCoefficients/fftROMindexing ==
  note: ROM is indexed by k=i-1 (zero offset)
      | so decrement by one.
  note: Determine when we transition to the
      | negative frequencies in the FFT frame
  note: Matlab FFT index i = 1:NFFT
  note: Matlab conjugate index = NFFT - i + 2
  note: Assert conjugation when counting through
      | the conjugate negative frequencies.
      | If we are dealing with negative frequencies
      | we need to know when to apply a
      | conjugation operation.
  note: Count from 1 to NFFT
      | while fftValid is asserted
  fftValid : Inport
  Add : Sum  Inputs=-+
  Bitwise Operator : simulink/Logic and Bit Operations/Bitwise Operator  logicop=NOT  UseBitMask=off  BitMask=bin2dec('11011001')  BitMaskRealWorld=Stored Integer
  Bitwise Operator1 : simulink/Logic and Bit Operations/Bitwise Operator  logicop=NOT  UseBitMask=off  BitMask=bin2dec('11011001')  BitMaskRealWorld=Stored Integer
  Constant1 : Constant  Value=modelParams.fft.size + 2  OutDataTypeStr=fixdt(0,modelParams.fft.Nbits+1,0)  SampleTime=modelParams.audio.samplePeriod/modelParams.system.upsampleFactor
  Constant5 : Constant  Value=modelParams.fft.sizeHalf+1  OutDataTypeStr=fixdt(0,modelParams.fft.Nbits,0)  SampleTime=modelParams.audio.samplePeriod/modelParams.system.upsampleFactor
  Decrement Stored Integer : hdlsllib/Math Operations/Decrement Stored Integer
  Relational Operator : RelationalOperator  Operator=<=  OutDataTypeStr=boolean  ZeroCross=off  InputSameDT=off
  Switch : Switch  Criteria=u2 > Threshold  SaturateOnIntegerOverflow=off  InputSameDT=off
  fftIndexCount : hdlsllib/Sources/HDL Counter  CountType=Free running  CountInit=0  CountStep=1  CountMax=25  CountFromType=Initial value  CountFrom=0  CountResetPort=on  CountLoadPort=off  CountEnbPort=on  CountDirPort=off  CountHitOutputPort=off  CountDataType=Unsigned  CountWordLen=modelParams.fft.Nbits+1  CountFracLen=0  CountSampTime=1
  ROMindex : Outport
  conjugate : Outport  Port=2
  wires:
  Bitwise Operator/1 -> fftIndexCount/1
  fftIndexCount/1 -> Add/1, Switch/1, Relational Operator/1
  fftValid/1 -> fftIndexCount/2, Bitwise Operator/1
  Constant5/1 -> Relational Operator/2
  Switch/1 -> Decrement Stored Integer/1
  Relational Operator/1 -> Switch/2, Bitwise Operator1/1
  Bitwise Operator1/1 -> conjugate/1
  Constant1/1 -> Add/2
  Add/1 -> Switch/3
  Decrement Stored Integer/1 -> ROMindex/1

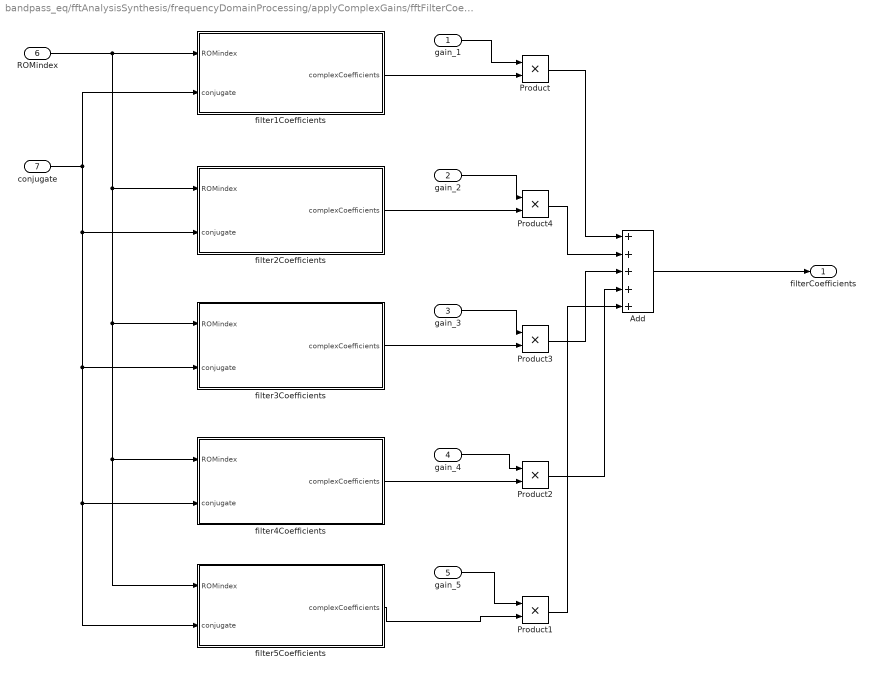
== system bandpass_eq/fftAnalysisSynthesis/frequencyDomainProcessing/applyComplexGains/fftFilterCoefficients/filterChoice ==
  gain_1 : Inport
  gain_2 : Inport  Port=2
  gain_3 : Inport  Port=3
  gain_4 : Inport  Port=4
  gain_5 : Inport  Port=5
  ROMindex : Inport  Port=6
  conjugate : Inport  Port=7
  Add : Sum  Inputs=+++++
  Product{,1..4} (5 alike) : Product
  filter1Coefficients : Subsystem
  filter2Coefficients : Subsystem
  filter3Coefficients : Subsystem
  filter4Coefficients : Subsystem
  filter5Coefficients : Subsystem
  filterCoefficients : Outport
  wires:
  ROMindex/1 -> filter5Coefficients/1(ROMindex), filter4Coefficients/1(ROMindex), filter3Coefficients/1(ROMindex), filter2Coefficients/1(ROMindex), filter1Coefficients/1(ROMindex)
  filter1Coefficients/1(complexCoefficients) -> Product/2
  conjugate/1 -> filter1Coefficients/2(conjugate), filter5Coefficients/2(conjugate), filter4Coefficients/2(conjugate), filter3Coefficients/2(conjugate), filter2Coefficients/2(conjugate)
  filter2Coefficients/1(complexCoefficients) -> Product4/2
  filter3Coefficients/1(complexCoefficients) -> Product3/2
  filter4Coefficients/1(complexCoefficients) -> Product2/2
  Product/1 -> Add/1
  Product4/1 -> Add/2
  Product3/1 -> Add/3
  Product2/1 -> Add/4
  Add/1 -> filterCoefficients/1
  filter5Coefficients/1(complexCoefficients) -> Product1/2
  Product1/1 -> Add/5
  gain_1/1 -> Product/1
  gain_2/1 -> Product4/1
  gain_3/1 -> Product3/1
  gain_4/1 -> Product2/1
  gain_5/1 -> Product1/1

== system bandpass_eq/fftAnalysisSynthesis/frequencyDomainProcessing/applyComplexGains/fftFilterCoefficients/filterChoice/filter1Coefficients ==
  note: The coefficients are only stored for the positive frequencies
      | The same coefficients are used for the negative frequencies but with a sign change.
  note: When conjugate is asserted
      | change the sign of the complex term.
  note: Perform conjuation of the imaginary term
      | for the negative frequencies
  ROMindex : Inport
  conjugate : Inport  Port=2
  Real-Imag to Complex : RealImagToComplex
  Switch : Switch  Criteria=u2 ~= 0  SaturateOnIntegerOverflow=off  InputSameDT=off
  Unary Minus : UnaryMinus
  filter1ImagCoefficients : LookupNDDirect  NumberOfTableDimensions=1  Table=modelParams.fftGainsF1Imag  TableDataTypeStr=modelParams.fftROMDataType
  filter1RealCoefficients : LookupNDDirect  NumberOfTableDimensions=1  Table=modelParams.fftGainsF1Real  TableDataTypeStr=modelParams.fftROMDataType
  complexCoefficients : Outport
  wires:
  ROMindex/1 -> filter1ImagCoefficients/1, filter1RealCoefficients/1
  filter1RealCoefficients/1 -> Real-Imag to Complex/1
  Real-Imag to Complex/1 -> complexCoefficients/1
  conjugate/1 -> Switch/2
  filter1ImagCoefficients/1 -> Unary Minus/1, Switch/3
  Switch/1 -> Real-Imag to Complex/2
  Unary Minus/1 -> Switch/1

== system bandpass_eq/fftAnalysisSynthesis/frequencyDomainProcessing/applyComplexGains/fftFilterCoefficients/filterChoice/filter2Coefficients ==
  note: Perform conjuation of the imaginary term
      | for the negative frequencies
  note: When conjugate is asserted
      | change the sign of the complex term.
  note: The coefficients are only stored for the positive frequencies
      | The same coefficients are used for the negative frequencies but with a sign change.
  ROMindex : Inport
  conjugate : Inport  Port=2
  Real-Imag to Complex : RealImagToComplex
  Switch1 : Switch  Criteria=u2 ~= 0  SaturateOnIntegerOverflow=off  InputSameDT=off
  Unary Minus : UnaryMinus
  filter2ImagCoefficients : LookupNDDirect  NumberOfTableDimensions=1  Table=modelParams.fftGainsF2Imag  TableDataTypeStr=modelParams.fftROMDataType
  filter2RealCoefficients : LookupNDDirect  NumberOfTableDimensions=1  Table=modelParams.fftGainsF2Real  TableDataTypeStr=modelParams.fftROMDataType
  complexCoefficients : Outport
  wires:
  ROMindex/1 -> filter2ImagCoefficients/1, filter2RealCoefficients/1
  filter2ImagCoefficients/1 -> Unary Minus/1, Switch1/3
  Switch1/1 -> Real-Imag to Complex/2
  Unary Minus/1 -> Switch1/1
  conjugate/1 -> Switch1/2
  filter2RealCoefficients/1 -> Real-Imag to Complex/1
  Real-Imag to Complex/1 -> complexCoefficients/1

== system bandpass_eq/fftAnalysisSynthesis/frequencyDomainProcessing/applyComplexGains/fftFilterCoefficients/filterChoice/filter3Coefficients ==
  note: Perform conjuation of the imaginary term
      | for the negative frequencies
  note: When conjugate is asserted
      | change the sign of the complex term.
  note: The coefficients are only stored for the positive frequencies
      | The same coefficients are used for the negative frequencies but with a sign change.
  ROMindex : Inport
  conjugate : Inport  Port=2
  Real-Imag to Complex : RealImagToComplex
  Switch1 : Switch  Criteria=u2 ~= 0  SaturateOnIntegerOverflow=off  InputSameDT=off
  Unary Minus : UnaryMinus
  filter3ImagCoefficients : LookupNDDirect  NumberOfTableDimensions=1  Table=modelParams.fftGainsF3Imag  TableDataTypeStr=modelParams.fftROMDataType
  filter3RealCoefficients : LookupNDDirect  NumberOfTableDimensions=1  Table=modelParams.fftGainsF3Real  TableDataTypeStr=modelParams.fftROMDataType
  complexCoefficients : Outport
  wires:
  ROMindex/1 -> filter3ImagCoefficients/1, filter3RealCoefficients/1
  filter3ImagCoefficients/1 -> Unary Minus/1, Switch1/3
  Switch1/1 -> Real-Imag to Complex/2
  Unary Minus/1 -> Switch1/1
  conjugate/1 -> Switch1/2
  filter3RealCoefficients/1 -> Real-Imag to Complex/1
  Real-Imag to Complex/1 -> complexCoefficients/1

== system bandpass_eq/fftAnalysisSynthesis/frequencyDomainProcessing/applyComplexGains/fftFilterCoefficients/filterChoice/filter4Coefficients ==
  note: Perform conjuation of the imaginary term
      | for the negative frequencies
  note: When conjugate is asserted
      | change the sign of the complex term.
  note: The coefficients are only stored for the positive frequencies
      | The same coefficients are used for the negative frequencies but with a sign change.
  note: The coefficients are only stored for the positive frequencies
      | The same coefficients are used for the negative frequencies but with a sign change.
  note: The coefficients are only stored for the positive frequencies
      | The same coefficients are used for the negative frequencies but with a sign change.
  ROMindex : Inport
  conjugate : Inport  Port=2
  Real-Imag to Complex : RealImagToComplex
  Switch1 : Switch  Criteria=u2 ~= 0  SaturateOnIntegerOverflow=off  InputSameDT=off
  Unary Minus : UnaryMinus
  filter4ImagCoefficients1 : LookupNDDirect  NumberOfTableDimensions=1  Table=modelParams.fftGainsF4Imag  TableDataTypeStr=modelParams.fftROMDataType
  filter4RealCoefficients1 : LookupNDDirect  NumberOfTableDimensions=1  Table=modelParams.fftGainsF4Real  TableDataTypeStr=modelParams.fftROMDataType
  complexCoefficients : Outport
  wires:
  ROMindex/1 -> filter4ImagCoefficients1/1, filter4RealCoefficients1/1
  filter4ImagCoefficients1/1 -> Unary Minus/1, Switch1/3
  Switch1/1 -> Real-Imag to Complex/2
  Unary Minus/1 -> Switch1/1
  conjugate/1 -> Switch1/2
  filter4RealCoefficients1/1 -> Real-Imag to Complex/1
  Real-Imag to Complex/1 -> complexCoefficients/1

== system bandpass_eq/fftAnalysisSynthesis/frequencyDomainProcessing/applyComplexGains/fftFilterCoefficients/filterChoice/filter5Coefficients ==
  note: The coefficients are only stored for the positive frequencies
      | The same coefficients are used for the negative frequencies but with a sign change.
  note: When conjugate is asserted
      | change the sign of the complex term.
  note: Perform conjuation of the imaginary term
      | for the negative frequencies
  ROMindex : Inport
  conjugate : Inport  Port=2
  Real-Imag to Complex : RealImagToComplex
  Switch : Switch  Criteria=u2 ~= 0  SaturateOnIntegerOverflow=off  InputSameDT=off
  Unary Minus : UnaryMinus
  filter1ImagCoefficients : LookupNDDirect  NumberOfTableDimensions=1  Table=modelParams.fftGainsF5Imag  TableDataTypeStr=modelParams.fftROMDataType
  filter1RealCoefficients : LookupNDDirect  NumberOfTableDimensions=1  Table=modelParams.fftGainsF5Real  TableDataTypeStr=modelParams.fftROMDataType
  complexCoefficients : Outport
  wires:
  ROMindex/1 -> filter1ImagCoefficients/1, filter1RealCoefficients/1
  filter1RealCoefficients/1 -> Real-Imag to Complex/1
  Real-Imag to Complex/1 -> complexCoefficients/1
  conjugate/1 -> Switch/2
  filter1ImagCoefficients/1 -> Unary Minus/1, Switch/3
  Switch/1 -> Real-Imag to Complex/2
  Unary Minus/1 -> Switch/1

== matlab function bandpass_eq/fftAnalysisSynthesis/analysis/fftFrameBuffering/addrBgen/addrBStateMachine ==
  data: powerup output; start input; frameShiftCounterEnable output; fftIndexCounterReset output; fftIndexCounterEnable output; fftCountHit input; fftValid output
function [powerup, frameShiftCounterEnable, fftIndexCounterReset, fftIndexCounterEnable, fftValid]  = addrB_state_machine(start, fftCountHit)
%#codegen


%-----------------------------------------------------------
% States
%-----------------------------------------------------------
state_powerup   = fi(0, 0, 3, 0);  % initialization state
state_wait      = fi(1, 0, 3, 0);  % wait for start pulse
state_counting  = fi(2, 0, 3, 0);  % counting state
state_count_end = fi(3, 0, 3, 0);  % counting state
state_update    = fi(4, 0, 3, 0);  % update the frame shift counter

persistent current_state;
if isempty(current_state)
    current_state = state_powerup;
end

%-----------------------------------------------------------
% default control values
%-----------------------------------------------------------
powerup                 = false;
frameShiftCounterEnable = false;
fftIndexCounterReset    = true;
fftIndexCounterEnable   = false;
fftValid                = false;

%-----------------------------------------------------------
% State machine for counter control signals
%-----------------------------------------------------------
switch(current_state)
    %-------------------------------------------------------
    case state_powerup  % wait for start pulse

        powerup = true;

        current_state = state_wait;

    %-------------------------------------------------------
    case state_wait  % wait for start pulse

        if start == 1
            current_state = state_counting;
        else
            current_state = state_wait;
        end
        
    %-------------------------------------------------------
    case state_counting % count from 0 to FFT length
        
        fftIndexCounterReset  = false;
        fftIndexCounterEnable = true;
        fftValid              = true;
              
        if fftCountHit == 1
            current_state = state_update;
        else
            current_state = state_counting;
        end
        
    %-------------------------------------------------------
    case state_count_end % count from 0 to FFT length
        
        fftIndexCounterReset  = false;
        fftIndexCounterEnable = true;
        fftValid              = true;
              
        current_state = state_update;
        
    %-------------------------------------------------------
    case state_update
        
        fftIndexCounterReset    = false;
        frameShiftCounterEnable = true;
        
        current_state = state_wait;
        
    otherwise
        
        current_state = state_powerup;
end

== matlab function bandpass_eq/fftAnalysisSynthesis/synthesis/overlapAdd/fifoStateMachine2 ==
  data: valid input; pop output
function pop = fifoStateMachine(valid)
%#codegen

stateValidLow        = fi(0, 0, 2, 0);
stateValidHigh       = fi(1, 0, 2, 0);
stateAssertPopSignal = fi(2, 0, 2, 0);

persistent current_state;
if isempty(current_state)
    current_state = stateValidLow;  % start in the low state
end

switch(current_state)
    case stateValidLow  % what for iFFTValid signal to be asserted for the first time

        pop = false;
        
        if valid
            current_state = stateValidHigh;
        else
            current_state = stateValidLow;
        end
        
    case stateValidHigh  % wait until the iFFTValid signal is deasserted
        
        pop = false;
        
        if valid
            current_state = stateValidHigh; 
        else
            current_state = stateAssertPopSignal;
        end
        
    case stateAssertPopSignal % assert pop signal forever after first iFFTValid signal
        
        pop = true;
        
        current_state = stateAssertPopSignal;
        
    otherwise
        
        pop = false;
        
end

== matlab function bandpass_eq/fftAnalysisSynthesis/synthesis/overlapAdd/fifoStateMachine3 ==
  data: valid input; pop output
function pop = fifoStateMachine(valid)
%#codegen

stateValidLow        = fi(0, 0, 2, 0);
stateValidHigh       = fi(1, 0, 2, 0);
stateAssertPopSignal = fi(2, 0, 2, 0);

persistent current_state;
if isempty(current_state)
    current_state = stateValidLow;  % start in the low state
end

switch(current_state)
    case stateValidLow  % what for iFFTValid signal to be asserted for the first time

        pop = false;
        
        if valid
            current_state = stateValidHigh;
        else
            current_state = stateValidLow;
        end
        
    case stateValidHigh  % wait until the iFFTValid signal is deasserted
        
        pop = false;
        
        if valid
            current_state = stateValidHigh; 
        else
            current_state = stateAssertPopSignal;
        end
        
    case stateAssertPopSignal % assert pop signal forever after first iFFTValid signal
        
        pop = true;
        
        current_state = stateAssertPopSignal;
        
    otherwise
        
        pop = false;
        
end

== matlab function bandpass_eq/fftAnalysisSynthesis/synthesis/overlapAdd/fifoStateMachine4 ==
  data: valid input; pop output
function pop = fifoStateMachine(valid)
%#codegen

stateValidLow        = fi(0, 0, 2, 0);
stateValidHigh       = fi(1, 0, 2, 0);
stateAssertPopSignal = fi(2, 0, 2, 0);

persistent current_state;
if isempty(current_state)
    current_state = stateValidLow;  % start in the low state
end

switch(current_state)
    case stateValidLow  % what for iFFTValid signal to be asserted for the first time

        pop = false;
        
        if valid
            current_state = stateValidHigh;
        else
            current_state = stateValidLow;
        end
        
    case stateValidHigh  % wait until the iFFTValid signal is deasserted
        
        pop = false;
        
        if valid
            current_state = stateValidHigh; 
        else
            current_state = stateAssertPopSignal;
        end
        
    case stateAssertPopSignal % assert pop signal forever after first iFFTValid signal
        
        pop = true;
        
        current_state = stateAssertPopSignal;
        
    otherwise
        
        pop = false;
        
end

== matlab function bandpass_eq/fftAnalysisSynthesis/synthesis/overlapAdd/fifoWriteSelect ==
  data: fifoCounter input; valid1 output; validSignal input; valid2 output; valid3 output; valid4 output
function [valid1, valid2, valid3, valid4] = fifoSelect(fifoCounter, validSignal)
%#codegen

switch fifoCounter
    case 0
        valid1 = validSignal;
        valid2 = false;
        valid3 = false;
        valid4 = false;
    case 1
        valid1 = false;
        valid2 = validSignal;
        valid3 = false;
        valid4 = false;
    case 2
        valid1 = false;
        valid2 = false;
        valid3 = validSignal;
        valid4 = false;
    case 3
        valid1 = false;
        valid2 = false;
        valid3 = false;
        valid4 = validSignal;
    otherwise
        valid1 = false;
        valid2 = false;
        valid3 = false;
        valid4 = false;
       
end

== matlab function bandpass_eq/fftAnalysisSynthesis/synthesis/overlapAdd/fifoStateMachine1 ==
  data: valid input; pop output
function pop = fifoStateMachine(valid)
%#codegen

stateValidLow        = fi(0, 0, 2, 0);
stateValidHigh       = fi(1, 0, 2, 0);
stateAssertPopSignal = fi(2, 0, 2, 0);

persistent current_state;
if isempty(current_state)
    current_state = stateValidLow;  % start in the low state
end

switch(current_state)
    case stateValidLow  % what for iFFTValid signal to be asserted for the first time

        pop = false;
        
        if valid
            current_state = stateValidHigh;
        else
            current_state = stateValidLow;
        end
        
    case stateValidHigh  % wait until the iFFTValid signal is deasserted
        
        pop = false;
        
        if valid
            current_state = stateValidHigh; 
        else
            current_state = stateAssertPopSignal;
        end
        
    case stateAssertPopSignal % assert pop signal forever after first iFFTValid signal
        
        pop = true;
        
        current_state = stateAssertPopSignal;
        
    otherwise
        
        pop = false;
        
end
